simulink model "HSMC_pendubot_simulation"  (Simulink 9.3)
settings: Solver=ode3  StartTime=0.0  StopTime=5  FixedStep=0.01  RelTol=1e-3  EnableMultiTasking=on
undefined symbols (not defined in the file): a, c1, c2, k2, nuy2
settings Model: Creator=donghai  LastModifiedBy=User2
settings DataIOCC: LimitDataPoints=on  SignalLoggingSaveFormat=Dataset
settings OptimizationCC: ExpressionDepthLimit=2147483647
settings DebuggingCC: SolverPrmCheckMsg=warning  FcnCallInpInsideContextMsg=error  StateNameClashWarn=warning
settings GRTTargetCC: GeneratePreprocessorConditionals=Disable all  CombineOutputUpdateFcns=on  GRTInterface=off

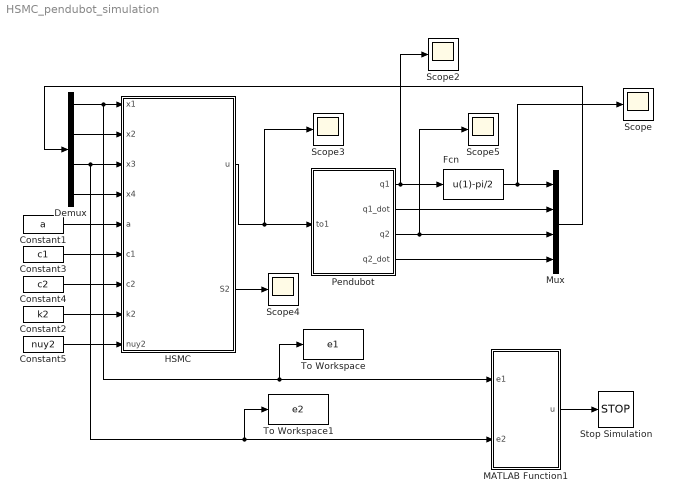
== system HSMC_pendubot_simulation ==
  Constant1 : Constant  Value=a
  Constant2 : Constant  Value=k2
  Constant3 : Constant  Value=c1
  Constant4 : Constant  Value=c2
  Constant5 : Constant  Value=nuy2
  Demux : Demux
  Fcn : Fcn  Expr=u(1)-pi/2
  "HSMC " : MATLAB Function  TreatAsAtomicUnit=on
  MATLAB Function1 : MATLAB Function  TreatAsAtomicUnit=on
  Mux : Mux
  Pendubot : Subsystem
  Scope{,2..5} (5 alike) : Scope
  Stop Simulation : Stop
  To Workspace : ToWorkspace  VariableName=e1  SampleTime=-1
  To Workspace1 : ToWorkspace  VariableName=e2  SampleTime=-1
  wires:
  "HSMC "/1(u) -> Scope3/1, Pendubot/1(to1)
  Pendubot/1(q1) -> Scope2/1, Fcn/1
  Demux/1 -> To Workspace/1, MATLAB Function1/1(e1), "HSMC "/1(x1)
  Demux/2 -> "HSMC "/2(x2)
  Demux/3 -> "HSMC "/3(x3), MATLAB Function1/2(e2), To Workspace1/1
  Demux/4 -> "HSMC "/4(x4)
  Fcn/1 -> Scope/1, Mux/1
  Pendubot/2(q1_dot) -> Mux/2
  Pendubot/3(q2) -> Scope5/1, Mux/3
  Pendubot/4(q2_dot) -> Mux/4
  Mux/1 -> Demux/1
  Constant1/1 -> "HSMC "/5(a)
  Constant3/1 -> "HSMC "/6(c1)
  Constant4/1 -> "HSMC "/7(c2)
  Constant2/1 -> "HSMC "/8(k2)
  Constant5/1 -> "HSMC "/9(nuy2)
  MATLAB Function1/1(u) -> Stop Simulation/1
  "HSMC "/2(S2) -> Scope4/1

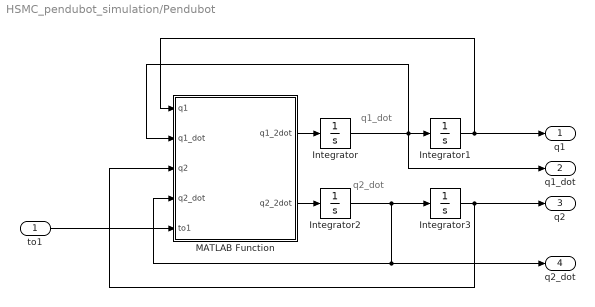
== system HSMC_pendubot_simulation/Pendubot ==
  note: q2_dot
  note: q1_dot
  to1 : Inport
  Integrator : Integrator
  Integrator1 : Integrator  InitialCondition=-pi/2
  Integrator2 : Integrator
  Integrator3 : Integrator
  MATLAB Function : MATLAB Function  TreatAsAtomicUnit=on
  q1 : Outport
  q1_dot : Outport  Port=2
  q2 : Outport  Port=3
  q2_dot : Outport  Port=4
  wires:
  MATLAB Function/1(q1_2dot) -> Integrator/1
  Integrator/1 -> MATLAB Function/2(q1_dot), q1_dot/1, Integrator1/1
  Integrator1/1 -> MATLAB Function/1(q1), q1/1
  MATLAB Function/2(q2_2dot) -> Integrator2/1
  Integrator2/1 -> MATLAB Function/4(q2_dot), q2_dot/1, Integrator3/1
  Integrator3/1 -> q2/1, MATLAB Function/3(q2)
  to1/1 -> MATLAB Function/5(to1)

== matlab function HSMC  ==
  data: u output double; x1 input double; x2 input double; x3 input double; x4 input double; a input double; c1 input double; c2 input double; k2 input double; nuy2 input double; S2 output double
function [u,S2] = fcn(x1,x2,x3,x4,a,c1,c2,k2,nuy2)
%% Declaration
beta1= 0.0308;
beta2= 0.0106;
beta3= 0.0095;
beta4= 0.2086;
beta5= 0.0630;
g=9.81;

%% DESIGN OF HIERARCHICAL SLIDING MODE CONTROL
f1=1/(beta1*beta2-beta3^2*(cos(x3))^2)*(beta2*beta3*(x2+x4)^2*sin(x3)+beta3^2*x2^2*sin(x3)*cos(x3)-beta2*beta4*g*cos((x1+pi/2))+beta3*beta5*g*cos(x3)*cos((x1+pi/2)+x3));
f2=1/(beta1*beta2-beta3^2*(cos(x3))^2)*(-beta3*(beta2+beta3*cos(x3))*(x2+x4)^2*sin(x3)-beta5*g*(beta1+beta3*cos(x3))*cos((x1+pi/2)+x3)+beta4*g*(beta2+beta3*cos(x3))*cos((x1+pi/2))-beta3*x2^2*sin(x3)*(beta1+beta3*cos(x3)));

b1 = beta2/(beta1*beta2 - beta3^2*cos(x3)^2);
b2 =(-beta2 - beta3*cos(x3))/(beta1*beta2 - beta3^2*cos(x3)^2);

%% Sliding mode surface
s1=c1*x1+x2;
s2=c2*x3+x4; 
S1=s1;
S2=a*S1+s2;

%% Equivalent control laws
u_eq_1=-(c1*x2+f1)/b1;
u_eq_2=-(c2*x4+f2)/b2;

%% Control input
u=((a*b1*u_eq_1+b2*u_eq_2)-(k2*S2+nuy2*sign(S2)))/(a*b1+b2);

== matlab function Pendubot/MATLAB Function ==
  data: q1 input double; q1_2dot output double; q1_dot input double; q2 input double; q2_dot input double; to1 input double; q2_2dot output double
function [q1_2dot,q2_2dot] = fcn(q1, q1_dot,q2,q2_dot,to1)
%% Declaration
beta1= 0.0308;
beta2= 0.0106;
beta3= 0.0095;
beta4= 0.2086;
beta5= 0.0630;
g=9.81;
%% Simulation
q1_2dot=1/(beta1*beta2-beta3^2*(cos(q2))^2)*(beta2*to1+beta2*beta3*(q1_dot+q2_dot)^2*sin(q2)+beta3^2*q1_dot^2*sin(q2)*cos(q2)-beta2*beta4*g*cos(q1)+beta3*beta5*g*cos(q2)*cos(q1+q2));
q2_2dot=1/(beta1*beta2-beta3^2*(cos(q2))^2)*((-beta2-beta3*cos(q2))*to1-beta3*(beta2+beta3*cos(q2))*(q1_dot+q2_dot)^2*sin(q2)-beta5*g*(beta1+beta3*cos(q2))*cos(q1+q2)+beta4*g*(beta2+beta3*cos(q2))*cos(q1)-beta3*q1_dot^2*sin(q2)*(beta1+beta3*cos(q2)));

== matlab function MATLAB Function1 ==
  data: u output double; e1 input double; e2 input double
function u  = fcn(e1,e2)
if ((abs(e1)>5)||(abs(e2)>5))
    u=1;
else
    u=0;
end
